simulink model "rx_dma_test"  (R2024a)
settings: Solver=FixedStepDiscrete  StartTime=0.0  StopTime=2e-3  RelTol=1e-3  EnableMultiTasking=on
PreLoadFcn:
  | ldcr_hdl_init();
InitFcn:
  | ldcr_hdl_init();
model workspace (MAT data in the model file):
  socvcb = containers.Map
  socvcb.serialization.keys = {}
  socvcb.serialization.values = {}
  socvcb.serialization.uniformity = 0
  socvcb.serialization.keyType = 'double'
  socvcb.serialization.valueType = 'any'
libraries: dspsrcs4 x2, dsphdlfiltering2 x2, simulink x2, hdlsllib x1
Description:
  | libiioSDRPSP_filter_example
  | 
  | A simple example model to demonstrate the use of MATLAB I/O alongside
  | hardware/software co-design.
  | 
  | Implements AXI programmable gain and bypassable filters on the Tx and Rx
  | paths of the HDL DUT.
settings Model: DataTypeOverride=Off  SimulationMode=accelerator  ExtModeTrigDuration=100  Creator=mfornero  LastModifiedBy=versal
settings SolverCC: AlgebraicLoopSolver=TrustRegion  PositivePriorityOrder=on  MaxZcPerStep=1
settings DataIOCC: SaveOutput=off  ReturnWorkspaceOutputs=off  StateSaveName=tmp_raccel_xout  SignalLoggingName=tmp_raccel_logsout
settings OptimizationCC: BlockReduction=off  ConditionallyExecuteInputs=off  DefaultParameterBehavior=Inlined  EnhancedBackFolding=on  PassReuseOutputArgsAs=Individual arguments  ZeroExternalMemoryAtStartup=off  ZeroInternalMemoryAtStartup=off  EfficientMapNaN2IntZero=off  MaxStackSize=64  OptimizeBlockOrder=speed  DifferentSizesBufferReuse=on  OptimizationCustomize=off  EfficientTunableParamExpr=on
settings DebuggingCC: AlgebraicLoopMsg=error  SingleTaskRateTransMsg=error  ParameterTunabilityLossMsg=error  UnconnectedInputMsg=warning  UnconnectedOutputMsg=warning  UnconnectedLineMsg=warning  PregeneratedLibrarySubsystemCodeDiagnostic=none  StrictBusMsg=ErrorOnBusTreatedAsVector  SFUnexpectedBacktrackingDiag=warning  SFNoUnconditionalDefaultTransitionDiag=warning  SFExecutionAtInitializationDiag=none  ArithmeticOperatorsInVariantConditions=warning
settings HardwareCC: ProdBitPerPointer=32  ProdBitPerSizeT=32  ProdBitPerPtrDiffT=32  ProdLargestAtomicFloat=None  ProdIntDivRoundTo=Undefined  ProdEndianess=Unspecified  ProdWordSize=32  ProdHWDeviceType=ASIC/FPGA->ASIC/FPGA  TargetBitPerLong=64  TargetBitPerPointer=64  TargetBitPerSizeT=64  TargetBitPerPtrDiffT=64  TargetLongLongMode=on  TargetIntDivRoundTo=Zero  TargetEndianess=LittleEndian  TargetWordSize=64  TargetHWDeviceType=Custom Processor->MATLAB Host Computer  ProdEqTarget=off  HardwareBoardFeatureSet=SoCBlockset
settings ModelReferenceCC: EnableRefExpFcnMdlSchedulingChecks=on  ModelReferenceNumInstancesAllowed=Single
settings SFSimCC: SimUseLocalCustomCode=off  CustomCodeUndefinedFunction=UseInterfaceOnly
settings RTWCC: Description=Embedded Coder  SystemTargetFile=ert.tlc  HardwareBoard=Custom Hardware Board  TLCOptions="-aInlineSetEventsForThisBaseRateFcn=TLC_FALSE -aSuppressMultiTaskScheduler=TLC_FALSE  -aRateBasedStepFcn=0"  TemplateMakefile=ert_default_tmf  RTWVerbose=off  RTWUseLocalCustomCode=off  RTWUseSimCustomCode=on  GPUComputeCapability=3.5  DLArmComputeVersion=19.05
settings CodeAppCC: ForceParamTrailComments=on  IgnoreCustomStorageClasses=off  MaxIdLength=128  OperatorAnnotations=on  SimulinkDataObjDesc=on  SFDataObjDesc=on  MangleLength=10  InsertBlockDesc=on
settings ERTTargetCC: InlinedParameterPlacement=NonHierarchical
settings ConfigComp: CovMetricSettings=dw  CovSaveCumulativeToWorkspaceVar=on  CovSaveSingleToWorkspaceVar=on  CovExternalEMLEnable=off

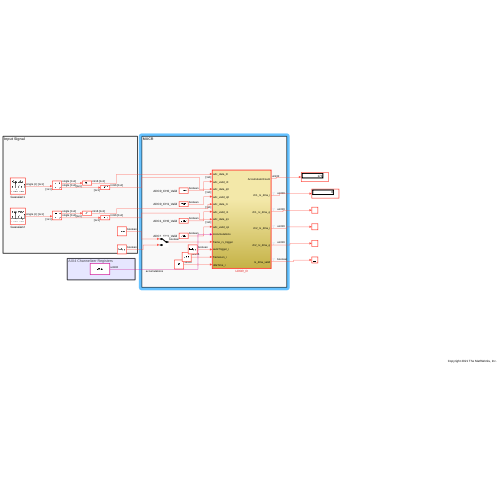
[thumbnail: Simulink's stored preview of the top-level diagram]
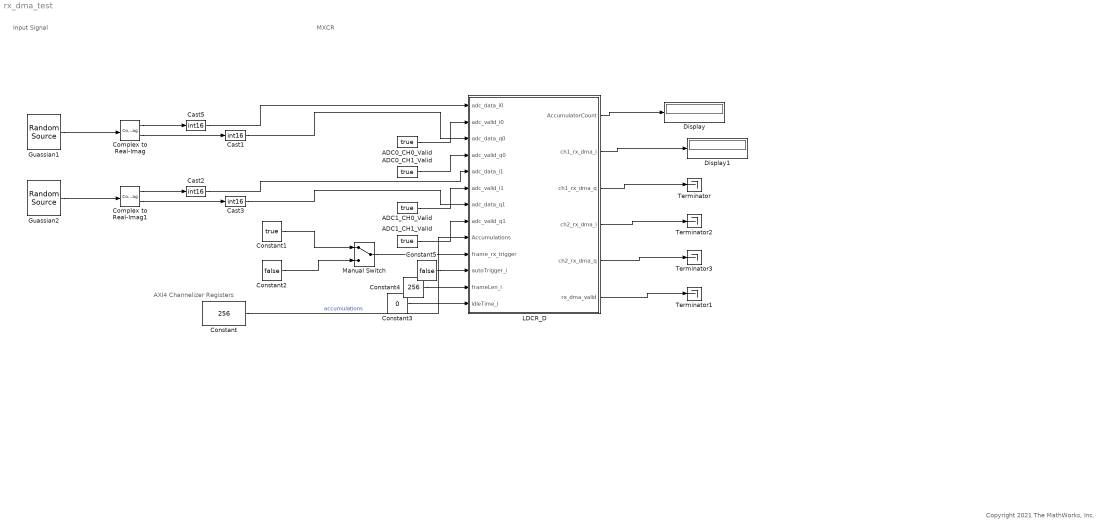
== system rx_dma_test ==
  note: AXI4 Channelizer Registers
  note: Copyright 2021 The MathWorks, Inc.
  note: MXCR
  note: Input Signal
  ADC0_CH0_Valid : Constant  Value=true  SampleTime=-1
  ADC0_CH1_Valid : Constant  Value=true  SampleTime=-1
  ADC1_CH0_Valid : Constant  Value=true  SampleTime=-1
  ADC1_CH1_Valid : Constant  Value=true  SampleTime=-1
  Cast{1..3,5} (4 alike) : DataTypeConversion  OutDataTypeStr=int16  SaturateOnIntegerOverflow=off  RndMeth=Floor
  Complex to Real-Imag : ComplexToRealImag
  Complex to Real-Imag1 : ComplexToRealImag
  Constant : Constant  Value=256  OutDataTypeStr=uint32
  Constant1 : Constant  Value=true  SampleTime=-1
  Constant2 : Constant  Value=false  SampleTime=-1
  Constant3 : Constant  Value=0  OutDataTypeStr=fixdt(1,24,0)  SampleTime=-1
  Constant4 : Constant  Value=256  OutDataTypeStr=uint16  SampleTime=-1
  Constant5 : Constant  Value=false  SampleTime=-1
  Display : Display
  Display1 : Display
  Guassian1 : dspsrcs4/Random Source  SrcType=Gaussian  MinVal=0  MaxVal=1  MeanVal=9  VarVal=24^2  RepMode=Specify seed  rawSeed=6547597  IsInherit=off  SampTime=Ts  SampFrame=1  OutComplex=Complex  DataType=single  SimulateUsing=Interpreted execution
  Guassian2 : dspsrcs4/Random Source  SrcType=Gaussian  MinVal=0  MaxVal=1  MeanVal=7  VarVal=24^2  RepMode=Specify seed  rawSeed=1324634  IsInherit=off  SampTime=Ts  SampFrame=1  OutComplex=Complex  DataType=single  SimulateUsing=Interpreted execution
  LDCR_D : Subsystem  TreatAsAtomicUnit=on
  Manual Switch : ManualSwitch
  Terminator{,1..3} (4 alike) : Terminator
  wires:
  ADC0_CH0_Valid/1 -> LDCR_D/2(adc_valid_i0)
  Constant/1 -> LDCR_D/9(Accumulations)  "accumulations"
  ADC0_CH1_Valid/1 -> LDCR_D/4(adc_valid_q0)
  ADC1_CH0_Valid/1 -> LDCR_D/6(adc_valid_i1)
  ADC1_CH1_Valid/1 -> LDCR_D/8(adc_valid_q1)
  Manual Switch/1 -> LDCR_D/10(frame_rx_trigger)
  LDCR_D/2(ch1_rx_dma_i) -> Display1/1
  LDCR_D/1(AccumulatorCount) -> Display/1
  Complex to Real-Imag/1 -> Cast5/1
  Complex to Real-Imag/2 -> Cast1/1
  Complex to Real-Imag1/1 -> Cast2/1
  Complex to Real-Imag1/2 -> Cast3/1
  Cast5/1 -> LDCR_D/1(adc_data_i0)
  Cast1/1 -> LDCR_D/3(adc_data_q0)
  Cast2/1 -> LDCR_D/5(adc_data_i1)
  Cast3/1 -> LDCR_D/7(adc_data_q1)
  Guassian1/1 -> Complex to Real-Imag/1
  Guassian2/1 -> Complex to Real-Imag1/1
  LDCR_D/3(ch1_rx_dma_q) -> Terminator/1
  LDCR_D/6(rx_dma_valid) -> Terminator1/1
  LDCR_D/4(ch2_rx_dma_i) -> Terminator2/1
  LDCR_D/5(ch2_rx_dma_q) -> Terminator3/1
  Constant1/1 -> Manual Switch/1
  Constant2/1 -> Manual Switch/2
  Constant3/1 -> LDCR_D/13(idleTime_i)
  Constant4/1 -> LDCR_D/12(frameLen_i)
  Constant5/1 -> LDCR_D/11(autoTrigger_i)

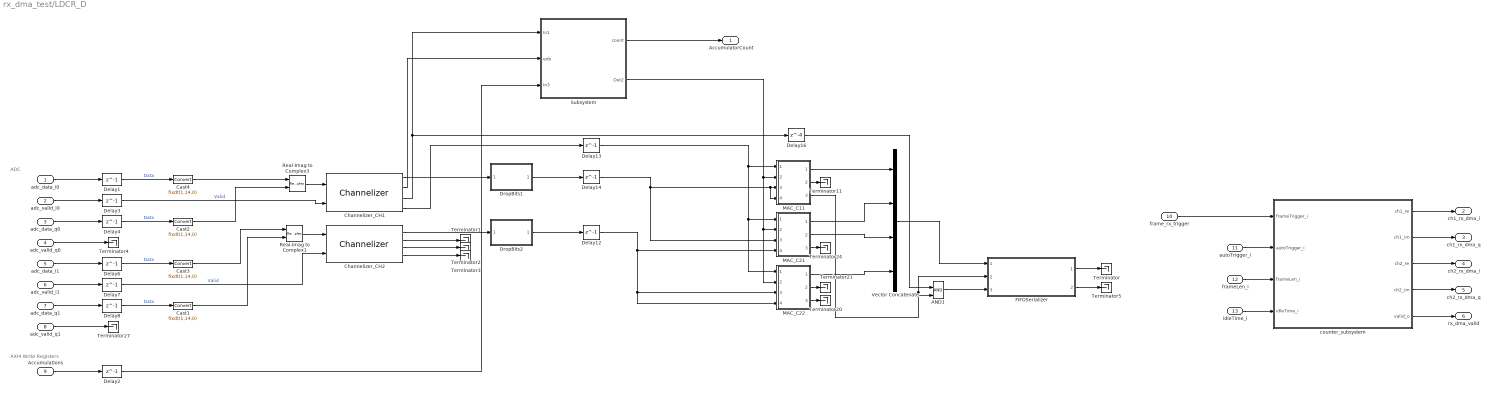
== system rx_dma_test/LDCR_D ==
  note: AXI4 Write Registers
  note: ADC
  adc_data_i0 : Inport
  adc_valid_i0 : Inport  Port=2
  adc_data_q0 : Inport  Port=3
  adc_valid_q0 : Inport  Port=4
  adc_data_i1 : Inport  Port=5
  adc_valid_i1 : Inport  Port=6
  adc_data_q1 : Inport  Port=7
  adc_valid_q1 : Inport  Port=8
  Accumulations : Inport  Port=9
  frame_rx_trigger : Inport  Port=10
  autoTrigger_i : Inport  Port=11
  frameLen_i : Inport  Port=12
  idleTime_i : Inport  Port=13
  AND1 : Logic  IconShape=distinctive  AllPortsSameDT=off  OutDataTypeStr=boolean
  Cast{1..4} (4 alike) : DataTypeConversion  OutDataTypeStr=fixdt(1,14,0)  SaturateOnIntegerOverflow=off  RndMeth=Floor
  Channelizer_CH1 : dsphdlfiltering2/Channelizer  FilterCoefficients=pfb.coeffs.Numerator  FilterStructure=Direct form systolic  NumFrequencyBands=fftsize  ComplexMultiplication=Use 3 multipliers and 5 adders  Normalize=off  OutputSize=Same as input size  SimulateUsing=Code generation  roundingMode=Floor  overflowMode=off  CoefficientsDataTypeStr=Inherit: Same word length as input  FilterOutputDataTypeStr=Inherit: Same word length as input  ResetInputPort=off  StartOutputPort=on  EndOutputPort=on
  Channelizer_CH2 : dsphdlfiltering2/Channelizer  FilterCoefficients=pfb.coeffs.Numerator  FilterStructure=Direct form systolic  NumFrequencyBands=fftsize  ComplexMultiplication=Use 3 multipliers and 5 adders  Normalize=off  OutputSize=Same as input size  SimulateUsing=Code generation  roundingMode=Floor  overflowMode=off  CoefficientsDataTypeStr=Inherit: Same word length as input  FilterOutputDataTypeStr=Inherit: Same word length as input  ResetInputPort=off  StartOutputPort=on  EndOutputPort=on
  Delay{1..4,6..8} (7 alike) : Delay  DelayLength=1
  Delay12 : Delay  DelayLength=1  InitialCondition=0  UseCircularBuffer=on
  Delay13 : Delay  DelayLength=1  InitialCondition=0  UseCircularBuffer=on
  Delay14 : Delay  DelayLength=1  InitialCondition=0  UseCircularBuffer=on
  Delay16 : Delay  DelayLength=4  InitialCondition=0  UseCircularBuffer=on
  DropBits1 : Subsystem  ReferencedSubsystem=DropBits
  DropBits2 : Subsystem  ReferencedSubsystem=DropBits
  FIFOSerializer : Subsystem  ReferencedSubsystem=FIFO_Serializer  FIFOLength=70
  MAC_C11 : Subsystem  ReferencedSubsystem=MAC
  MAC_C21 : Subsystem  ReferencedSubsystem=MAC
  MAC_C22 : Subsystem  ReferencedSubsystem=MAC
  Real-Imag to Complex1 : RealImagToComplex
  Real-Imag to Complex3 : RealImagToComplex
  Subsystem : Subsystem
  Terminator{,1..5,11,20..21,24,27} (11 alike) : Terminator
  Vector Concatenate : Concatenate  NumInputs=4
  counter_subsystem : Subsystem
  AccumulatorCount : Outport  VectorParamsAs1DForOutWhenUnconnected=off
  ch1_rx_dma_i : Outport  Port=2  VectorParamsAs1DForOutWhenUnconnected=off
  ch1_rx_dma_q : Outport  Port=3
  ch2_rx_dma_i : Outport  Port=4  VectorParamsAs1DForOutWhenUnconnected=off
  ch2_rx_dma_q : Outport  Port=5
  rx_dma_valid : Outport  Port=6
  wires:
  adc_data_i0/1 -> Delay1/1
  adc_valid_i0/1 -> Delay3/1
  Delay1/1 -> Cast4/1  "Data"
  Accumulations/1 -> Delay2/1
  adc_data_q0/1 -> Delay4/1
  adc_valid_q0/1 -> Terminator4/1
  adc_data_i1/1 -> Delay6/1
  adc_valid_i1/1 -> Delay7/1
  adc_data_q1/1 -> Delay8/1
  adc_valid_q1/1 -> Terminator27/1
  Delay4/1 -> Cast2/1  "Data"
  Delay6/1 -> Cast3/1  "Data"
  Delay8/1 -> Cast1/1  "Data"
  Delay16/1 -> AND1/1
  Delay14/1 -> MAC_C21/3, MAC_C11/3, MAC_C11/4
  Delay12/1 -> MAC_C22/4, MAC_C22/3, MAC_C21/4
  MAC_C22/1 -> Vector Concatenate/4
  MAC_C21/2 -> Vector Concatenate/3
  MAC_C21/1 -> Vector Concatenate/2
  MAC_C11/1 -> Vector Concatenate/1
  MAC_C21/3 -> Terminator24/1
  MAC_C22/2 -> Terminator21/1
  MAC_C22/3 -> Terminator20/1
  MAC_C11/2 -> Terminator11/1
  Delay13/1 -> MAC_C22/1, MAC_C21/1, MAC_C11/1
  Channelizer_CH2/4 -> Terminator3/1
  Channelizer_CH2/3 -> Terminator2/1
  Channelizer_CH2/2 -> Terminator1/1
  Vector Concatenate/1 -> FIFOSerializer/1
  Channelizer_CH1/4 -> Delay13/1
  Channelizer_CH1/3 -> Subsystem/1(In1), Delay16/1
  MAC_C11/3 -> FIFOSerializer/2, AND1/2
  AND1/1 -> FIFOSerializer/3
  Channelizer_CH2/1 -> DropBits2/1
  Channelizer_CH1/1 -> DropBits1/1
  DropBits1/1 -> Delay14/1
  DropBits2/1 -> Delay12/1
  Real-Imag to Complex1/1 -> Channelizer_CH2/1
  Real-Imag to Complex3/1 -> Channelizer_CH1/1
  Cast1/1 -> Real-Imag to Complex1/2
  Cast3/1 -> Real-Imag to Complex1/1
  Cast2/1 -> Real-Imag to Complex3/2
  Cast4/1 -> Real-Imag to Complex3/1
  Delay3/1 -> Channelizer_CH1/2  "Valid"
  Delay7/1 -> Channelizer_CH2/2  "Valid"
  FIFOSerializer/1 -> Terminator/1
  FIFOSerializer/2 -> Terminator5/1
  Subsystem/2(Out2) -> MAC_C22/2, MAC_C21/2, MAC_C11/2
  Channelizer_CH1/2 -> Subsystem/2(enb)
  Delay2/1 -> Subsystem/3(In3)
  Subsystem/1(count) -> AccumulatorCount/1
  frame_rx_trigger/1 -> counter_subsystem/1(frameTrigger_i)
  counter_subsystem/1(ch1_re) -> ch1_rx_dma_i/1
  counter_subsystem/2(ch1_im) -> ch1_rx_dma_q/1
  counter_subsystem/3(ch2_re) -> ch2_rx_dma_i/1
  counter_subsystem/4(ch2_im) -> ch2_rx_dma_q/1
  counter_subsystem/5(valid_o) -> rx_dma_valid/1
  autoTrigger_i/1 -> counter_subsystem/2(autoTrigger_i)
  frameLen_i/1 -> counter_subsystem/3(frameLen_i)
  idleTime_i/1 -> counter_subsystem/4(idleTime_i)

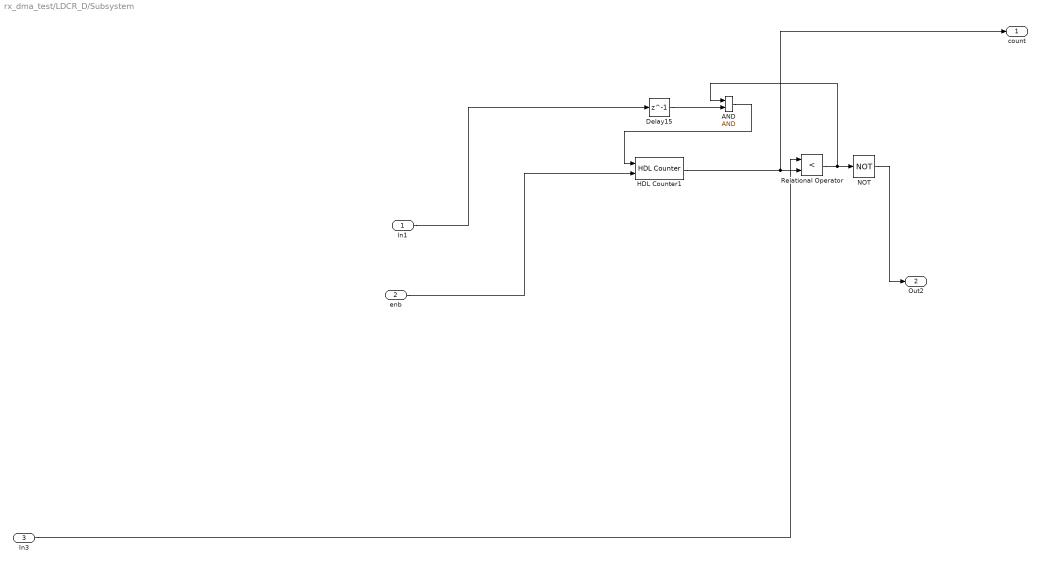
== system rx_dma_test/LDCR_D/Subsystem ==
  In1 : Inport
  enb : Inport  Port=2
  In3 : Inport  Port=3
  AND : Logic  IconShape=distinctive  AllPortsSameDT=off  OutDataTypeStr=boolean
  Delay15 : Delay  DelayLength=1  InitialCondition=0  UseCircularBuffer=on
  HDL Counter1 : hdlsllib/Sources/HDL Counter  CountType=Free running  CountInit=0  CountStep=1  CountMax=16  CountFromType=Initial value  CountFrom=0  CountResetPort=on  CountLoadPort=off  CountEnbPort=on  CountDirPort=off  CountHitOutputPort=off  CountDataType=Unsigned  CountWordLen=32  CountFracLen=0  CountSampTime=1
  NOT : Logic  Operator=NOT  IconShape=distinctive  AllPortsSameDT=off  OutDataTypeStr=boolean
  Relational Operator : RelationalOperator  Operator=<  OutDataTypeStr=boolean  RndMeth=Simplest  InputSameDT=off
  count : Outport
  Out2 : Outport  Port=2
  wires:
  AND/1 -> HDL Counter1/1
  Delay15/1 -> AND/2
  Relational Operator/1 -> AND/1, NOT/1
  NOT/1 -> Out2/1
  In3/1 -> Relational Operator/1
  In1/1 -> Delay15/1
  enb/1 -> HDL Counter1/2
  HDL Counter1/1 -> count/1, Relational Operator/2

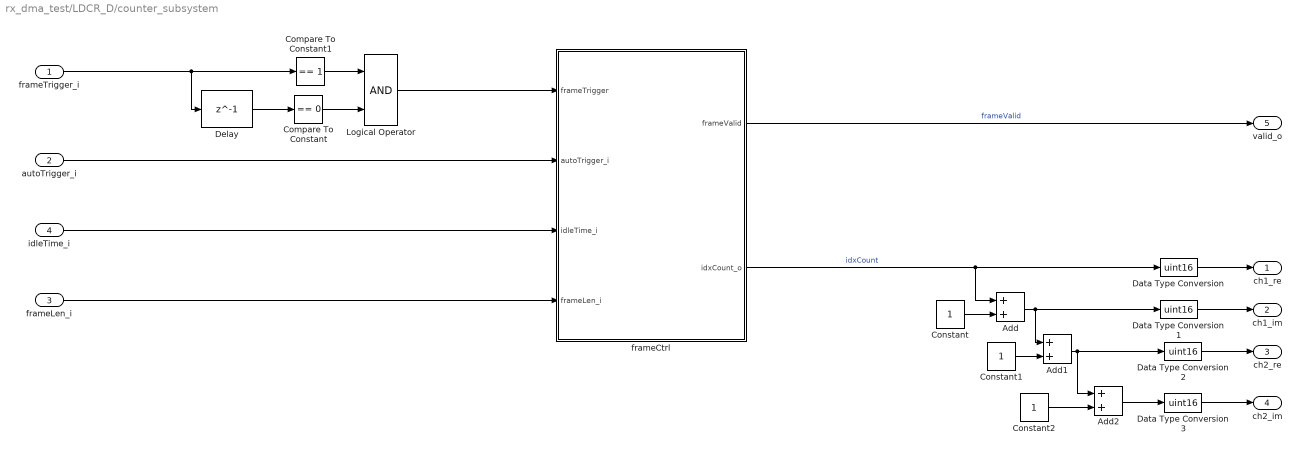
== system rx_dma_test/LDCR_D/counter_subsystem ==
  frameTrigger_i : Inport
  autoTrigger_i : Inport  Port=2
  frameLen_i : Inport  Port=3
  idleTime_i : Inport  Port=4
  Add : Sum
  Add1 : Sum
  Add2 : Sum
  Compare To Constant : simulink/Logic and Bit Operations/Compare To Constant  relop===  const=0  OutDataTypeStr=boolean
  Compare To Constant1 : simulink/Logic and Bit Operations/Compare To Constant  relop===  const=1  OutDataTypeStr=boolean
  Constant : Constant  OutDataTypeStr=uint16  SampleTime=-1
  Constant1 : Constant  OutDataTypeStr=uint16  SampleTime=-1
  Constant2 : Constant  OutDataTypeStr=uint16  SampleTime=-1
  Data Type Conversion{,1..3} (4 alike) : DataTypeConversion  OutDataTypeStr=uint16  SaturateOnIntegerOverflow=off  RndMeth=Floor
  Delay : Delay  DelayLength=1  InitialCondition=0  UseCircularBuffer=on
  Logical Operator : Logic  IconShape=distinctive  AllPortsSameDT=off  OutDataTypeStr=boolean
  frameCtrl : MATLAB Function  TreatAsAtomicUnit=on
  ch1_re : Outport
  ch1_im : Outport  Port=2
  ch2_re : Outport  Port=3
  ch2_im : Outport  Port=4
  valid_o : Outport  Port=5
  wires:
  Constant/1 -> Add/2
  Constant2/1 -> Add2/2
  Constant1/1 -> Add1/2
  Add/1 -> Data Type Conversion1/1, Add1/1
  Add2/1 -> Data Type Conversion3/1
  Add1/1 -> Data Type Conversion2/1, Add2/1
  Data Type Conversion1/1 -> ch1_im/1
  Data Type Conversion/1 -> ch1_re/1
  Data Type Conversion2/1 -> ch2_re/1
  Data Type Conversion3/1 -> ch2_im/1
  frameLen_i/1 -> frameCtrl/4(frameLen_i)
  autoTrigger_i/1 -> frameCtrl/2(autoTrigger_i)
  Logical Operator/1 -> frameCtrl/1(frameTrigger)
  frameTrigger_i/1 -> Delay/1, Compare To Constant1/1
  Delay/1 -> Compare To Constant/1
  frameCtrl/1(frameValid) -> valid_o/1  "frameValid"
  frameCtrl/2(idxCount_o) -> Add/1, Data Type Conversion/1  "idxCount"
  Compare To Constant/1 -> Logical Operator/2
  Compare To Constant1/1 -> Logical Operator/1
  idleTime_i/1 -> frameCtrl/3(idleTime_i)

== matlab function rx_dma_test/LDCR_D/counter_subsystem/frameCtrl ==
  data: frameTrigger input; autoTrigger_i input; idleTime_i input; frameLen_i input; frameValid output; idxCount_o output
function [frameValid,idxCount_o] = frameControl(frameTrigger,autoTrigger_i,idleTime_i,frameLen_i)
persistent frameLenReg frameCtrlState autoTrigModeReg idxCount idleCount idleLength

FRAME_IDLE_TIME = 1024*10; % wait time in clock cycles - default value

S_TRIGGER_WAIT = fi(0,0,3,0);
S_FRAME_SEND   = fi(1,0,3,0);
S_FRAME_IDLE   = fi(2,0,3,0);

if isempty(frameLenReg)
    frameCtrlState = S_TRIGGER_WAIT;
    frameLenReg = uint16(1024); % default frame length value
    autoTrigModeReg = false;
    idxCount = uint16(0);
    idleCount = fi(0,0,24,0);
    idleLength = fi(FRAME_IDLE_TIME,0,24,0);
end

% y = u;
idxCount_o = idxCount;
frameValid = false;

switch(frameCtrlState)
    case(S_TRIGGER_WAIT)
  
        if (frameTrigger || autoTrigModeReg)
            frameCtrlState(:) = S_FRAME_SEND; % begin data send
        end

        % update registers
        if frameLen_i ~= 0
            frameLenReg(:) = frameLen_i; 
        end       
        autoTrigModeReg(:) = autoTrigger_i;
        if idleTime_i ~= 0
            idleLength(:)  = idleTime_i;
        end

    case(S_FRAME_SEND)
        if idxCount >= (frameLenReg - 1)  % last index in frame reached
            idxCount(:)    = 0;          % Reset index counter            
            frameCtrlState(:) = S_FRAME_IDLE;
        else
            idxCount(:) = idxCount  + 1;
        end
        frameValid = true;

    case(S_FRAME_IDLE)
        if idleCount >= (idleLength - 1) % reached last index
            idleCount(:) = 0;
            if autoTrigModeReg
                frameCtrlState(:) = S_FRAME_SEND;
            else
                frameCtrlState(:) = S_TRIGGER_WAIT;
            end
        else
           idleCount(:) = idleCount + 1;
        end
        frameLenReg(:)     = frameLen_i; % update registers. If on auto-trigger we want to make sure the length is updated
        autoTrigModeReg(:) = autoTrigger_i;

end
